simulink model "Qbot_2022a_standalone_odom"  (R2023a)
settings: Solver=ode1  StartTime=0.0  StopTime=inf  FixedStep=1/60  RelTol=1e-3
PostLoadFcn:
  | qlabs_setup
model workspace: external: MATLAB File Qbot_2022a_saveas.m (data not in the file)
values from neighbouring files (symbols this model uses):
  R = 0.04445    [param.m]
  Tinv = inv(T)    [param.m]
  X0 = [0 0 0]'    [param.m]
libraries: quarc_library x9, simulink x2
settings Model: SimulationMode=external  ExtModeTrigDuration=10000  Creator=mbohra  LastModifiedBy=surya
settings DebuggingCC: UnderspecifiedInitializationDetection=Classic  MergeDetectMultiDrivingBlocksExec=none
settings ModelReferenceCC: PropagateSignalLabelsOutOfModel=off

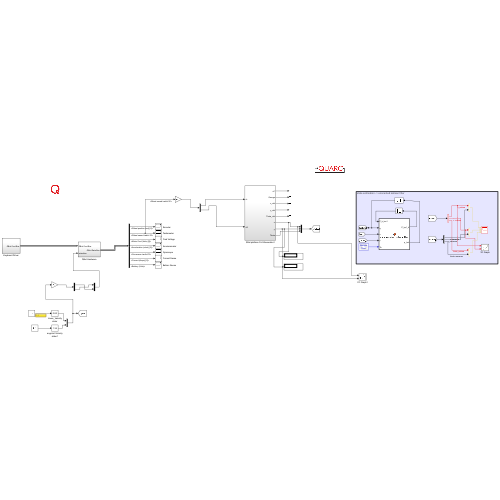
[thumbnail: Simulink's stored preview of the top-level diagram]
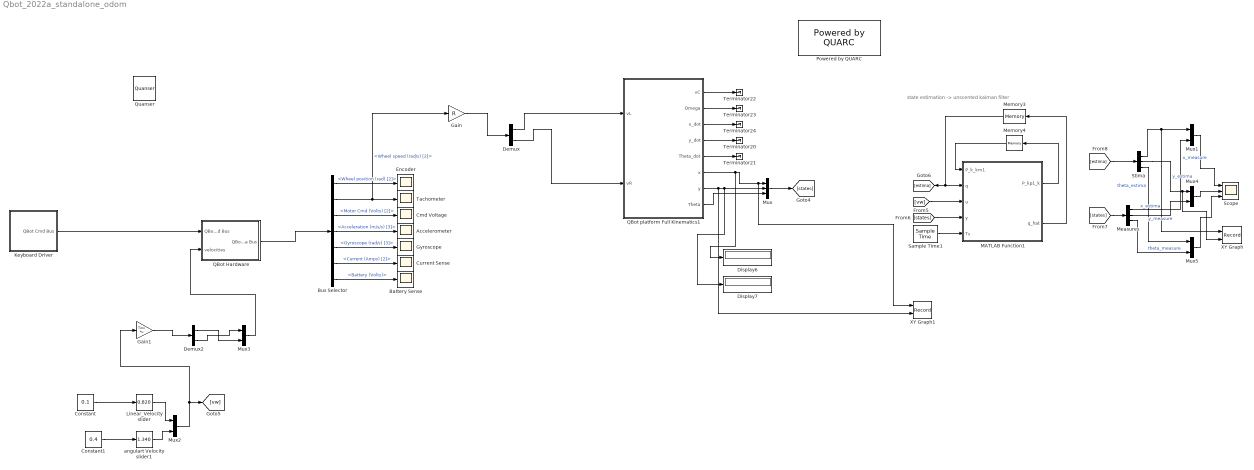
== system Qbot_2022a_standalone_odom ==
  note: state estimation -> unscented kalman filter
  Accelerometer : Scope
  Battery Sense : Scope
  Bus Selector : BusSelector  OutputSignals=Wheel position (rad) [2],Wheel speed (rad/s) [2],Motor Cmd (Volts) [2],Acceleration (m/s/s) [3],Gyroscope (rad/s) [3],Current (Amps) [2],Battery (Volts)
  Cmd Voltage : Scope
  Constant : Constant  Value=0.1
  Constant1 : Constant  Value=0.4
  Current Sense : Scope
  Demux : Demux  Outputs=2
  Demux2 : Demux  Outputs=2
  Display6 : Display
  Display7 : Display
  Encoder : Scope
  Gain : Gain  Gain=R
  Gain1 : Gain  Gain=Tinv  Multiplication=Matrix(K*u)
  Gyroscope : Scope
  Keyboard Driver : Subsystem
  Linear_Velocity slider : simulink/Math Operations/Slider Gain  gain=0.820  low=0  high=2
  MATLAB Function1 : MATLAB Function  TreatAsAtomicUnit=on
  Measures : Demux  Outputs=3
  Memory3 : Memory  InitialCondition=X0
  Memory4 : Memory  InitialCondition=1e-3*eye(3)
  Mux : Mux  Inputs=3
  Mux{1..5} (5 alike) : Mux  Inputs=2
  Powered by QUARC : quarc_library/Logos/Powered by QUARC
  QBot Hardware : Subsystem
  QBot platform Full Kinematics1 : Subsystem
  Quanser : quarc_library/Logos/Quanser
  Sample Time1 : quarc_library/Sources/Time/Sample Time  Priority=-99  sample_time=Ts
  Scope : Scope  NumInputPorts=3
  Stima : Demux  Outputs=3
  Tachometer : Scope
  Terminator{20..24} (5 alike) : Terminator
  XY Graph : Record  FileSettingsInternal="{\"entries\":[{\"content\":{\"excelSettings\":{\"content\":{},\"type\":\"Streamout.ExcelSettings\"}},\"type\":\"Streamout.FileSettingStorage\",\"uuid\":\"\"}],\"packageUris\":[\"http:\\/\\/schema.mathworks.com\\/mf0\\/streamout_blocks\\/R2020a\"],\"version\":\"1.0\"}"  Layout=[1 1]  SignalsInternal="{\"entries\":[{\"content\":{\"signals\":[{\"content\":{\"blockPath\":[],\"dimensions\":[1,1],\"domain\":\"\",\"lineColor\":\"#a2142f\",\"plots\":[1],\"port\":1,\"sid\":[\"\"],\"signalID\":12210,\"signalName\":\"x_estima\"},\"type\":\"RecordBlkView.Signal\",\"uuid\":\"\"},{\"content\":{\"blockPath\":[],\"dimensions\":[1,1],\"domain\":\"\",\"lineColor\":\"#139fff\",\"plots\":[1],\"port\":2,\"sid\":[\"\"],\"signalID\":12214,\"signalName\":\"y_estima\"},\"type\":\"RecordBlkView.Signal\",\"uuid\":\"\"}]},\"type\":\"RecordBlkView.InputSignals\",\"uuid\":\"\"}],\"packageUris\":[\"http:\\/\\/schema.mathworks.com\\/mf0\\/streamout_blocks\\/R2020a\"],\"version\":\"1.0\"}"  VisualizationBindings="{\"xyplotplugin\":{\"info\":[{\"series\":[{\"bindingParametersList\":[{\"parameter\":\"X-Axis\",\"signalID\":12210,\"signalName\":\"x_estima\"},{\"parameter\":\"Y-Axis\",\"signalID\":12214,\"signalName\":\"y_estima\"}],\"seriesID\":53143}],\"subplotID\":1}]}}"  CompatibilityTag=XY
  XY Graph1 : Record  FileSettingsInternal="{\"entries\":[{\"content\":{\"excelSettings\":{\"content\":{},\"type\":\"Streamout.ExcelSettings\"}},\"type\":\"Streamout.FileSettingStorage\",\"uuid\":\"\"}],\"packageUris\":[\"http:\\/\\/schema.mathworks.com\\/mf0\\/streamout_blocks\\/R2020a\"],\"version\":\"1.0\"}"  Layout=[1 1]  SignalsInternal="{\"entries\":[{\"content\":{\"signals\":[{\"content\":{\"blockPath\":[],\"dimensions\":[1],\"domain\":\"\",\"lineColor\":\"#0072bd\",\"port\":1,\"sid\":[\"\"],\"signalID\":12218,\"signalName\":\"QBot platform Full Kinematics1:6\"},\"type\":\"RecordBlkView.Signal\",\"uuid\":\"\"},{\"content\":{\"blockPath\":[],\"dimensions\":[1],\"domain\":\"\",\"lineColor\":\"#d95319\",\"port\":2,\"sid\":[\"\"],\"signalID\":12222,\"signalName\":\"QBot platform Full Kinematics1:7\"},\"type\":\"RecordBlkView.Signal\",\"uuid\":\"\"}]},\"type\":\"RecordBlkView.InputSignals\",\"uuid\":\"\"}],\"packageUris\":[\"http:\\/\\/schema.mathworks.com\\/mf0\\/streamout_blocks\\/R2020a\"],\"version\":\"1.0\"}"  VisualizationBindings="{\"xyplotplugin\":{\"info\":[{\"series\":[{\"bindingParametersList\":[{\"parameter\":\"X-Axis\",\"signalID\":7088,\"signalName\":\"reference_trajectory1:1\"},{\"parameter\":\"Y-Axis\",\"signalID\":7092,\"signalName\":\"reference_trajectory1:2\"}],\"seriesID\":58991}],\"subplotID\":1}]}}"  CompatibilityTag=XY
  angulart Velocity slider1 : simulink/Math Operations/Slider Gain  gain=1.340  low=0  high=2
  wires:
  Bus Selector/7 -> Battery Sense/1  "<Battery (Volts)>"
  Keyboard Driver/1(QBot Cmd Bus) -> QBot Hardware/1(QBot Cmd Bus)
  Bus Selector/1 -> Encoder/1  "<Wheel position (rad) [2]>"
  Bus Selector/3 -> Cmd Voltage/1  "<Motor Cmd (Volts) [2]>"
  Bus Selector/4 -> Accelerometer/1  "<Acceleration (m/s/s) [3]>"
  QBot Hardware/1(QBot Data Bus) -> Bus Selector/1
  Bus Selector/6 -> Current Sense/1  "<Current (Amps) [2]>"
  Bus Selector/5 -> Gyroscope/1  "<Gyroscope (rad/s) [3]>"
  Demux/2 -> QBot platform Full Kinematics1/2(vR)
  QBot platform Full Kinematics1/4(y_dot) -> Terminator20/1
  Demux/1 -> QBot platform Full Kinematics1/1(vL)
  QBot platform Full Kinematics1/6(x) -> XY Graph1/1, Mux/1, Display6/1
  QBot platform Full Kinematics1/8(Theta) -> Mux/3
  Mux/1 -> [states]
  QBot platform Full Kinematics1/2(Omega) -> Terminator23/1
  QBot platform Full Kinematics1/7(y) -> Mux/2, Display7/1, XY Graph1/2
  QBot platform Full Kinematics1/1(vC) -> Terminator22/1
  QBot platform Full Kinematics1/3(x_dot) -> Terminator24/1
  QBot platform Full Kinematics1/5(Theta_dot) -> Terminator21/1
  Gain/1 -> Demux/1
  Bus Selector/2 -> Gain/1, Tachometer/1  "<Wheel speed (rad/s) [2]>"
  MATLAB Function1/1(P_kp1_k) -> Memory4/1
  [states] -> MATLAB Function1/4(y)
  Stima/3 -> Mux5/1  "theta_estima"
  MATLAB Function1/2(q_hat) -> Memory3/1
  Sample Time1/1 -> MATLAB Function1/5(Ts)
  Stima/2 -> XY Graph/2, Mux4/1  "y_estima"
  Measures/1 -> Mux1/2  "x_measure"
  Measures/2 -> Mux4/2  "y_measure"
  Mux1/1 -> Scope/1
  Memory3/1 -> MATLAB Function1/2(q), [estima]
  Mux5/1 -> Scope/3
  Mux4/1 -> Scope/2
  [states] -> Measures/1
  Measures/3 -> Mux5/2  "theta_measure"
  Stima/1 -> XY Graph/1, Mux1/1  "x_estima"
  [vw] -> MATLAB Function1/3(u)
  [estima] -> Stima/1
  Memory4/1 -> MATLAB Function1/1(P_k_km1)
  Gain1/1 -> Demux2/1
  Demux2/1 -> Mux3/2
  Demux2/2 -> Mux3/1
  Mux3/1 -> QBot Hardware/2(velocities)
  Constant/1 -> Linear_Velocity slider/1
  Constant1/1 -> angulart Velocity slider1/1
  Linear_Velocity slider/1 -> Mux2/1
  angulart Velocity slider1/1 -> Mux2/2
  Mux2/1 -> Gain1/1, [vw]

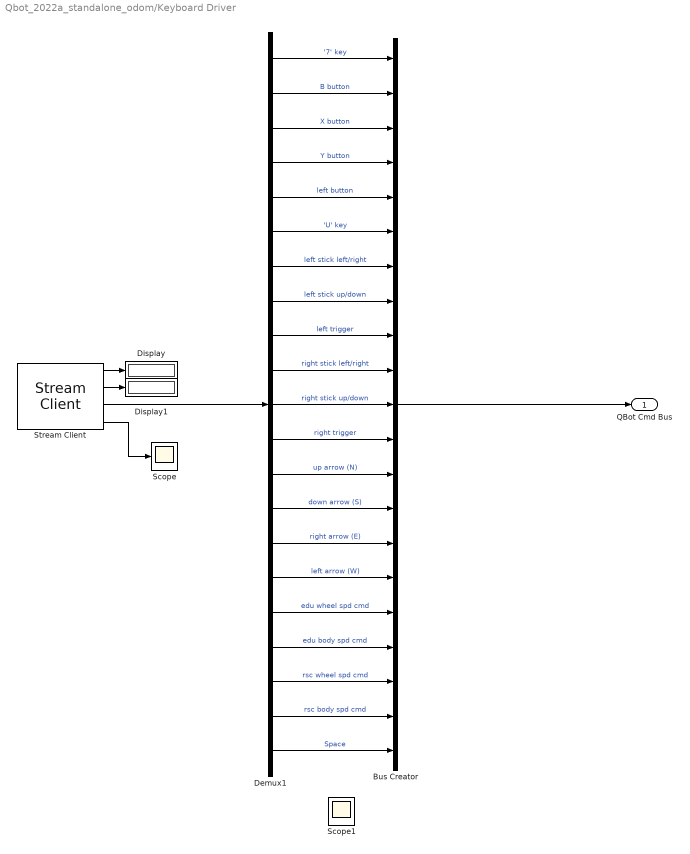
== system Qbot_2022a_standalone_odom/Keyboard Driver ==
  Bus Creator : BusCreator  Inputs=21
  Demux1 : Demux  Outputs=[1 1 1 1 1 1 1 1 1 1 1 1 1 1 1 1 2 2 2 2 1]
  Display : Display
  Display1 : Display
  Scope : Scope
  Scope1 : Scope
  Stream Client : quarc_library/Communications/Basic/Stream Client  uri_source=Specify via dialog (do not evaluate)  uri=tcpip://localhost:18889?nagle='off'  send_buffer_size=1460  receive_buffer_size=1460  byte_order=little endian (Intel - LSB first)  optimization=Minimum latency  send_options=Do not send data  receive_options=Receive most recent data  default_value=zeros(25,1)  sample_time=qc_get_step_size  active=on  implementation=Use blocking I/O in a separate thread  send_fifo_size=1000  receive_fifo_size=1000  send_priority=0  receive_priority=0  send_dimensions=off  receive_dimensions=off  max_dimensions=-1  data_type=Inherited via back propagation  type_expr=BusObject
      settings: AttributesFormatString="\"tcpip://localhost:18889?nagle='off'\""
  QBot Cmd Bus : Outport
  wires:
  Bus Creator/1 -> QBot Cmd Bus/1
  Stream Client/3 -> Demux1/1
  Demux1/1 -> Bus Creator/1  "'7' key"
  Demux1/2 -> Bus Creator/2  "B button"
  Demux1/3 -> Bus Creator/3  "X button"
  Demux1/4 -> Bus Creator/4  "Y button"
  Demux1/5 -> Bus Creator/5  "left button"
  Demux1/6 -> Bus Creator/6  "'U' key"
  Demux1/7 -> Bus Creator/7  "left stick left/right"
  Demux1/8 -> Bus Creator/8  "left stick up/down"
  Demux1/9 -> Bus Creator/9  "left trigger"
  Demux1/10 -> Bus Creator/10  "right stick left/right"
  Demux1/11 -> Bus Creator/11  "right stick up/down"
  Demux1/12 -> Bus Creator/12  "right trigger"
  Demux1/13 -> Bus Creator/13  "up arrow (N)"
  Demux1/14 -> Bus Creator/14  "down arrow (S)"
  Demux1/15 -> Bus Creator/15  "right arrow (E)"
  Demux1/16 -> Bus Creator/16  "left arrow (W)"
  Demux1/17 -> Bus Creator/17  "edu wheel spd cmd"
  Demux1/18 -> Bus Creator/18  "edu body spd cmd"
  Demux1/19 -> Bus Creator/19  "rsc wheel spd cmd"
  Demux1/20 -> Bus Creator/20  "rsc body spd cmd"
  Demux1/21 -> Bus Creator/21  "Space"
  Stream Client/1 -> Display/1
  Stream Client/2 -> Display1/1
  Stream Client/4 -> Scope/1

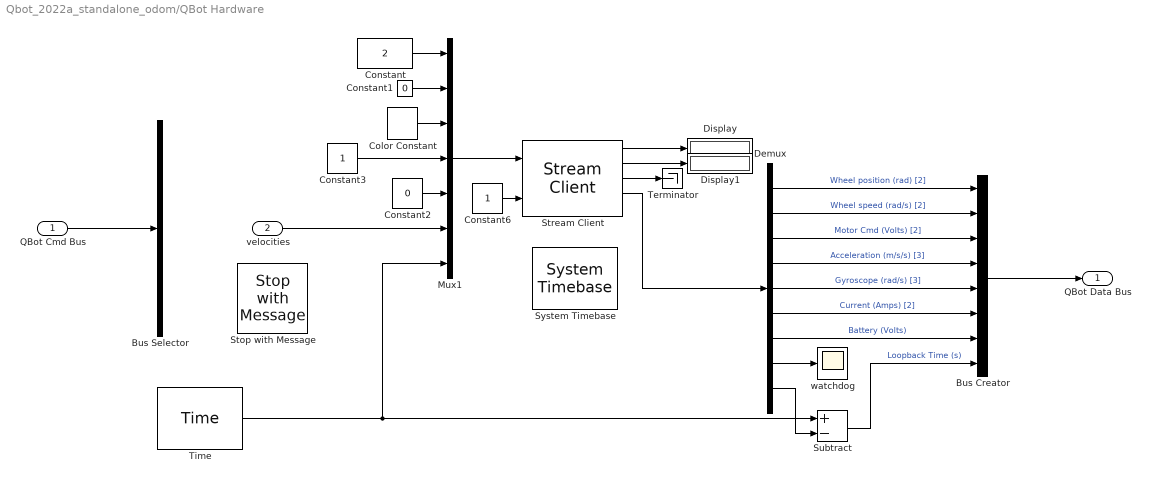
== system Qbot_2022a_standalone_odom/QBot Hardware ==
  QBot Cmd Bus : Inport
  velocities : Inport  Port=2
  Bus Creator : BusCreator  Inputs=8
  Bus Selector : BusSelector  OutputSignals=Space,edu body spd cmd,'U' key
  Color Constant : quarc_library/Sources/Signals/Color Constant  color=[0 1 1]
      settings: SourceProductName=QUARC Targets
  Constant : Constant  Value=2
  Constant1 : Constant  Value=0
  Constant2 : Constant  Value=0
  Constant3 : Constant
  Constant6 : Constant
  Demux : Demux  Outputs=[2 2 2 3 3 2 1 1 1]
  Display : Display
  Display1 : Display
  Mux1 : Mux  Inputs=7
  Stop with Message : quarc_library/Sinks/Error Handling/Stop with Message  message_type=Fixed error message  message_icon=Information  message=Operator: Emergency Stop
  Stream Client : quarc_library/Communications/Basic/Stream Client  uri_source=Specify via dialog (do not evaluate)  uri=tcpip://localhost:18888  send_buffer_size=1460  receive_buffer_size=1460  byte_order=little endian (Intel - LSB first)  optimization=Minimum latency  send_options=Send most recent data  receive_options=Receive most recent data  default_value=zeros(17,1)  sample_time=qc_get_step_size  active=on  implementation=Use blocking I/O in a separate thread  send_fifo_size=1000  receive_fifo_size=1000  send_priority=0  receive_priority=0  send_dimensions=off  receive_dimensions=off  max_dimensions=-1  data_type=Inherited via back propagation  type_expr=BusObject
      settings: AttributesFormatString="\"tcpip://localhost:18888\""
  Subtract : Sum  Inputs=+-
  System Timebase : quarc_library/Advanced/Timing/System Timebase  stop_on_overrun=off
      settings: SourceProductName=QUARC Targets
  Terminator : Terminator
  Time : quarc_library/Sources/Time/Time  time_source=Wall clock  sample_time=qc_get_step_size
  watchdog : Scope
  QBot Data Bus : Outport
  wires:
  Demux/2 -> Bus Creator/2  "Wheel speed (rad/s) [2]"
  Constant/1 -> Mux1/1
  Stream Client/3 -> Terminator/1
  Stream Client/1 -> Display/1
  Constant6/1 -> Stream Client/2
  Stream Client/2 -> Display1/1
  Color Constant/1 -> Mux1/3
  Constant1/1 -> Mux1/2
  Demux/3 -> Bus Creator/3  "Motor Cmd (Volts) [2]"
  Mux1/1 -> Stream Client/1
  Stream Client/4 -> Demux/1
  Demux/1 -> Bus Creator/1  "Wheel position (rad) [2]"
  Demux/7 -> Bus Creator/7  "Battery (Volts)"
  Demux/5 -> Bus Creator/5  "Gyroscope (rad/s) [3]"
  Demux/6 -> Bus Creator/6  "Current (Amps) [2]"
  Demux/9 -> Subtract/2
  Constant2/1 -> Mux1/5
  Demux/4 -> Bus Creator/4  "Acceleration (m/s/s) [3]"
  Time/1 -> Subtract/1, Mux1/7
  Bus Creator/1 -> QBot Data Bus/1
  Subtract/1 -> Bus Creator/8  "Loopback Time (s)"
  Demux/8 -> watchdog/1
  QBot Cmd Bus/1 -> Bus Selector/1
  velocities/1 -> Mux1/6
  Constant3/1 -> Mux1/4

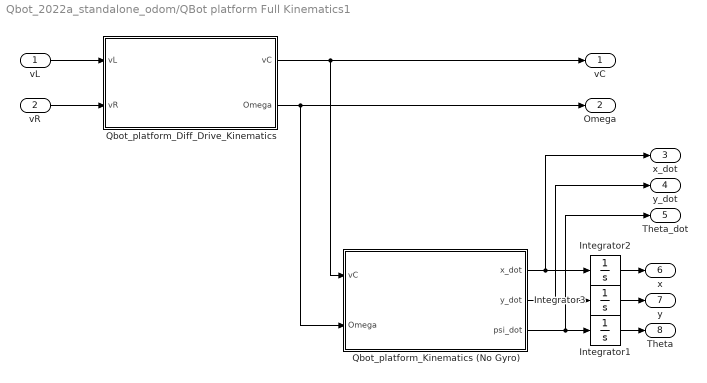
== system Qbot_2022a_standalone_odom/QBot platform Full Kinematics1 ==
  vL : Inport
  vR : Inport  Port=2
  Integrator1 : Integrator  InitialCondition=X0(3)
  Integrator2 : Integrator  InitialCondition=X0(1)
  Integrator3 : Integrator  InitialCondition=X0(2)
  Qbot_platform_Diff_Drive_Kinematics : Subsystem
  Qbot_platform_Kinematics (No Gyro) : Subsystem
  vC : Outport  VectorParamsAs1DForOutWhenUnconnected=off
  Omega : Outport  Port=2  VectorParamsAs1DForOutWhenUnconnected=off
  x_dot : Outport  Port=3  VectorParamsAs1DForOutWhenUnconnected=off
  y_dot : Outport  Port=4  VectorParamsAs1DForOutWhenUnconnected=off
  Theta_dot : Outport  Port=5  VectorParamsAs1DForOutWhenUnconnected=off
  x : Outport  Port=6  VectorParamsAs1DForOutWhenUnconnected=off
  y : Outport  Port=7  VectorParamsAs1DForOutWhenUnconnected=off
  Theta : Outport  Port=8  VectorParamsAs1DForOutWhenUnconnected=off
  wires:
  Integrator1/1 -> Theta/1
  Qbot_platform_Kinematics (No Gyro)/3(psi_dot) -> Theta_dot/1, Integrator1/1
  Qbot_platform_Kinematics (No Gyro)/1(x_dot) -> x_dot/1, Integrator2/1
  Qbot_platform_Kinematics (No Gyro)/2(y_dot) -> y_dot/1, Integrator3/1
  Qbot_platform_Diff_Drive_Kinematics/1(vC) -> Qbot_platform_Kinematics (No Gyro)/1(vC), vC/1
  vL/1 -> Qbot_platform_Diff_Drive_Kinematics/1(vL)
  vR/1 -> Qbot_platform_Diff_Drive_Kinematics/2(vR)
  Integrator2/1 -> x/1
  Integrator3/1 -> y/1
  Qbot_platform_Diff_Drive_Kinematics/2(Omega) -> Qbot_platform_Kinematics (No Gyro)/2(Omega), Omega/1

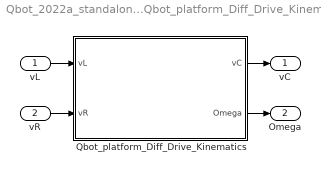
== system Qbot_2022a_standalone_odom/QBot platform Full Kinematics1/Qbot_platform_Diff_Drive_Kinematics ==
  vL : Inport
  vR : Inport  Port=2
  Qbot_platform_Diff_Drive_Kinematics : MATLAB Function  TreatAsAtomicUnit=on
  vC : Outport  VectorParamsAs1DForOutWhenUnconnected=off
  Omega : Outport  Port=2  VectorParamsAs1DForOutWhenUnconnected=off
  wires:
  vL/1 -> Qbot_platform_Diff_Drive_Kinematics/1(vL)
  Qbot_platform_Diff_Drive_Kinematics/1(vC) -> vC/1
  vR/1 -> Qbot_platform_Diff_Drive_Kinematics/2(vR)
  Qbot_platform_Diff_Drive_Kinematics/2(Omega) -> Omega/1

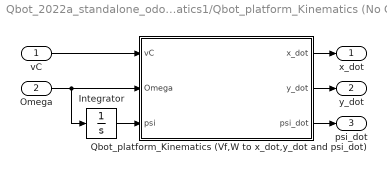
== system Qbot_2022a_standalone_odom/QBot platform Full Kinematics1/Qbot_platform_Kinematics (No Gyro) ==
  vC : Inport
  Omega : Inport  Port=2
  Integrator : Integrator
  Qbot_platform_Kinematics (Vf,W to x_dot,y_dot and psi_dot) : MATLAB Function  TreatAsAtomicUnit=on
  x_dot : Outport  VectorParamsAs1DForOutWhenUnconnected=off
  y_dot : Outport  Port=2  VectorParamsAs1DForOutWhenUnconnected=off
  psi_dot : Outport  Port=3  VectorParamsAs1DForOutWhenUnconnected=off
  wires:
  Qbot_platform_Kinematics (Vf,W to x_dot,y_dot and psi_dot)/3(psi_dot) -> psi_dot/1
  Integrator/1 -> Qbot_platform_Kinematics (Vf,W to x_dot,y_dot and psi_dot)/3(psi)
  vC/1 -> Qbot_platform_Kinematics (Vf,W to x_dot,y_dot and psi_dot)/1(vC)
  Qbot_platform_Kinematics (Vf,W to x_dot,y_dot and psi_dot)/1(x_dot) -> x_dot/1
  Omega/1 -> Integrator/1, Qbot_platform_Kinematics (Vf,W to x_dot,y_dot and psi_dot)/2(Omega)
  Qbot_platform_Kinematics (Vf,W to x_dot,y_dot and psi_dot)/2(y_dot) -> y_dot/1

== matlab function Qbot_2022a_standalone_odom/MATLAB Function1 ==
  data: P_k_km1 input; P_kp1_k output; q input; u input; q_hat output; y input; Ts input
function [P_kp1_k,q_hat]= my_unscented_kalman_filter(P_k_km1,q,u,y,Ts)
Q=1e-5*eye(3);
R=1e-4*eye(3);
alpha=0.9; beta=2; kappa=0;
%Calculate the Sigma points
M=3;
c=alpha^2*(M+kappa);
q_hat_i=zeros(M,2*M+1);
q_hat_i(:,1)=q;
Delta_x=real(sqrtm(c*P_k_km1));
for i=1:M
    q_hat_i(:,i+1)=q+Delta_x(:,i);
    q_hat_i(:,i+1+M)=q-Delta_x(:,i);
end
%Output of the sigma points
y_hat_i=q_hat_i(1:3,:);
%predicted measurement at time k
W_M=zeros(1,2*M+1);
W_M(1)=1-(M/(alpha^2*(M+kappa)));
W_M(2:2*M+1)=(1/(2*alpha^2*(M+kappa)));
y_k=zeros(3,1);
for i=1:2*M+1
    y_k=y_k+W_M(i)*y_hat_i(:,i);
end
%Estimate of the covariance of predicted measurement
W_c=zeros(1,2*M+1);
W_c(1)=(2-alpha^2+beta)-(M/(alpha^2*(M+kappa)));
W_c(2:2*M+1)=(1/(2*alpha^2*(M+kappa)));
P_y=zeros(3,3);
for i=1:2*M+1
    P_y=P_y+W_c(i)*(y_hat_i(:,i)-y_k)*(y_hat_i(:,i)-y_k)'+R;
end
%%Estimate of the cross-covariance between predicted x and y
P_xy=zeros(M,3);
for i=1:2*M+1
    P_xy=P_xy+(1/(2*alpha^2*(M+kappa)))*(q_hat_i(:,i)-q)*(y_hat_i(:,i)-y_k)';
end
%Kalman gain
K=P_xy/(P_y);
q_k_k = q+K*(y-y_k);
P_k_k = P_k_km1 -K*P_y*K';
% State prediction and state estimation error covariance
q_hat_i_k_k=zeros(M,2*M+1);
q_hat_i_k_k(:,1)=q_k_k;
Delta_x=real(sqrtm(c*P_k_k));
for i=1:M
    q_hat_i_k_k(:,i+1)=q_k_k+Delta_x(:,i);
    q_hat_i_k_k(:,i+1+M)=q_k_k-Delta_x(:,i);
end
%Predicted state for each sigma point
q_hat_kp1_k=zeros(M,2*M+1);
for i=1:2*M+1
    q_hat_kp1_k(:,i)=q_hat_i_k_k(:,i)+Ts*[cos(q_hat_i_k_k(3,i)) 0;
        sin(q_hat_i_k_k(3,i)) 0;
        0          1]*u;
end
%Predicted state k+1 at time k
q_hat=zeros(M,1);
for i=1:2*M+1
    q_hat=q_hat + W_M(i)*q_hat_kp1_k(:,i);
end
%Covariance of the predicted state
P_kp1_k=zeros(M,M);
for i=1:2*M+1
    P_kp1_k=P_kp1_k+W_c(i)*(q_hat_kp1_k(:,i)-q_hat)*(q_hat_kp1_k(:,i)-q_hat)'+Q;
end
end

== matlab function Qbot_2022a_standalone_odom/QBot platform Full Kinematics1/Qbot_platform_Diff_Drive_Kinematics/Qbot_platform_Diff_Drive_Kinematics ==
  data: vL input; vC output; vR input; Omega output
function [vC,Omega] = fcn(vL,vR)
%#codegen

d= 0.393;

vC=0.5*(vL+vR);
Omega=(1/d)*(vR-vL);

== matlab function Qbot_2022a_standalone_odom/QBot platform Full Kinematics1/Qbot_platform_Kinematics (No Gyro)/Qbot_platform_Kinematics (Vf,W to x_dot,y_dot and psi_dot) ==
  data: vC input; x_dot output; Omega input; y_dot output; psi input; psi_dot output
function [x_dot,y_dot,psi_dot] = fcn(vC,Omega,psi)
%#codegen


x_dot=cos(psi)*vC;
y_dot=sin(psi)*vC;
psi_dot= Omega;
